simulink model "Model_xspmono_csa_ga"  (R2017a)
settings: Solver=ode45  StartTime=4.3  StopTime=9.196  MaxStep=0.001  RelTol=1e-3  AbsTol=1e-3  EnableMultiTasking=on
values from neighbouring files (symbols this model uses):
  F1 = F(1:11)    [Plot_results_last.m]
  K1_csa_ga = 2.26205318539721    (= 2.2620531854)    [Plot_results_last.m]
  K5_csa_ga = 1.94337888356766    (= 1.94337888357)    [Plot_results_last.m]
  Ks_csa_ga = 0.00300000000000    (= 0.003)    [Plot_results_last.m]
  Mmax_csa_ga = 0.90000000000000    (= 0.9)    [Plot_results_last.m]
  P0 = P1(1)    [Plot_results_last.m]
  Sd = [Sdop; Sd1]    [Plot_results_last.m]
  So = 500    [Plot_results_last.m]
  t1 = t(1:11)    [Plot_results_last.m]
  V1 = V(1:11)    [Plot_results_last.m]
  Xd = [Xdop; Xd1]    [Plot_results_last.m]
settings Model: ExtModeTrigMode=oneshot  ExtModeArmWhenConnect=off  Creator=i7_Pc  LastModifiedBy=i7_Pc
settings DataIOCC: SaveFormat=Array  SignalLoggingSaveFormat=ModelDataLogs  SaveOutput=off  SaveTime=off
settings OptimizationCC: BlockReduction=off  BooleanDataType=off  ExpressionDepthLimit=2147483647  InitFltsAndDblsToZero=on  LifeSpan=inf
settings DebuggingCC: SaveWithParameterizedLinksMsg=none  UnderspecifiedInitializationDetection=Classic  MergeDetectMultiDrivingBlocksExec=none  SignalResolutionControl=TryResolveAllWithWarning  MultiTaskDSMMsg=warning  MultiTaskCondExecSysMsg=none  FcnCallInpInsideContextMsg=warning  StateNameClashWarn=warning  SFUnexpectedBacktrackingDiag=warning  SFNoUnconditionalDefaultTransitionDiag=warning  SFExecutionAtInitializationDiag=none
settings HardwareCC: ProdBitPerPointer=32  ProdBitPerSizeT=32  ProdBitPerPtrDiffT=32  ProdLargestAtomicFloat=None  ProdIntDivRoundTo=Undefined  ProdEndianess=Unspecified  ProdWordSize=32  ProdHWDeviceType=32-bit Generic  TargetUnknown=on
settings ModelReferenceCC: PropagateSignalLabelsOutOfModel=off
settings GRTTargetCC: TargetLangStandard=C89/C90 (ANSI)  GeneratePreprocessorConditionals=Disable all  CombineOutputUpdateFcns=off  GRTInterface=on
settings ConfigComp: CovMetricSettings=dw  CovHtmlReporting=on  CovSaveCumulativeToWorkspaceVar=on  CovSaveSingleToWorkspaceVar=on  CovExternalEMLEnable=off

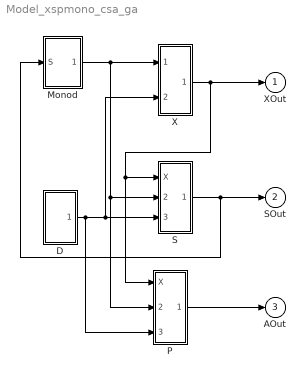
== system Model_xspmono_csa_ga ==
  D : Subsystem
  Monod : Subsystem
  P : Subsystem
  S : Subsystem
  X : Subsystem
  XOut : Outport
  SOut : Outport  Port=2
  AOut : Outport  Port=3
  wires:
  X/1(XOut) -> S/1(X), P/1(X), XOut/1
  S/1(Sout) -> Monod/1(S), SOut/1
  Monod/1(mu) -> X/1(mu), S/2(mu), P/2(mu)
  D/1(out_1) -> S/3(F/V), X/2(F/V), P/3(F/V)
  P/1(Pout) -> AOut/1

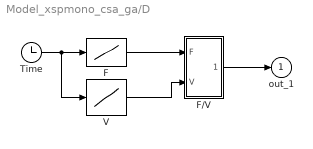
== system Model_xspmono_csa_ga/D ==
  F : Lookup  InputValues=t1  Table=F1  SaturateOnIntegerOverflow=on
  F/V : Subsystem  mask(/){}
      mask help: Division of two scalars. y=u[1]/u[2]
      mask Help: Division of two scalars: y=u[1]/u[2]
      mask Display: disp('/')
  Time : Clock
  V : Lookup  InputValues=t1  Table=V1  SaturateOnIntegerOverflow=on
  out_1 : Outport
  wires:
  F/V/1(out_1) -> out_1/1
  F/1 -> F/V/1(F)
  V/1 -> F/V/2(V)
  Time/1 -> F/1, V/1

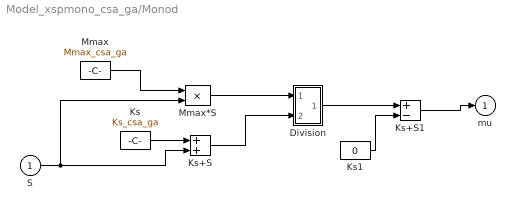
== system Model_xspmono_csa_ga/Monod ==
  S : Inport
  Division : Subsystem  mask(/){}
      mask help: Division of two scalars. y=u[1]/u[2]
      mask Help: Division of two scalars: y=u[1]/u[2]
      mask Display: disp('/')
  Ks : Constant  Value=Ks_csa_ga
  Ks+S : Sum  SaturateOnIntegerOverflow=on  InputSameDT=on  OutDataTypeStr=Inherit: Same as first input
  Ks+S1 : Sum  Inputs=+-  SaturateOnIntegerOverflow=on  InputSameDT=on  OutDataTypeStr=Inherit: Same as first input
  Ks1 : Constant  Value=0
  Mmax : Constant  Value=Mmax_csa_ga
  Mmax*S : Product  SaturateOnIntegerOverflow=on  RndMeth=Zero  InputSameDT=on  OutDataTypeStr=Inherit: Same as first input
  mu : Outport
  wires:
  Mmax/1 -> Mmax*S/1
  Mmax*S/1 -> Division/1(Mmax*S)
  Ks+S/1 -> Division/2(Ks+S)
  Ks/1 -> Ks+S/1
  S/1 -> Ks+S/2, Mmax*S/2
  Division/1(out_1) -> Ks+S1/1
  Ks1/1 -> Ks+S1/2
  Ks+S1/1 -> mu/1

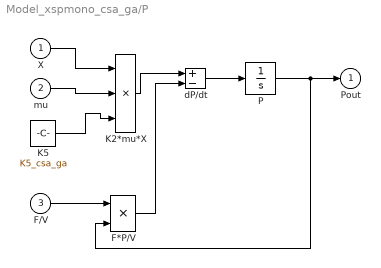
== system Model_xspmono_csa_ga/P ==
  X : Inport
  mu : Inport  Port=2
  F/V : Inport  Port=3
  F*P/V : Product  SaturateOnIntegerOverflow=on  RndMeth=Zero  InputSameDT=on  OutDataTypeStr=Inherit: Same as first input
  K2*mu*X : Product  Inputs=3  SaturateOnIntegerOverflow=on  RndMeth=Zero  InputSameDT=on  OutDataTypeStr=Inherit: Same as first input
  K5 : Constant  Value=K5_csa_ga
  P : Integrator  InitialCondition=P0
  dP/dt : Sum  Inputs=+-  SaturateOnIntegerOverflow=on  InputSameDT=on  OutDataTypeStr=Inherit: Same as first input
  Pout : Outport
  wires:
  P/1 -> Pout/1, F*P/V/2
  dP/dt/1 -> P/1
  K2*mu*X/1 -> dP/dt/1
  X/1 -> K2*mu*X/1
  mu/1 -> K2*mu*X/2
  F/V/1 -> F*P/V/1
  F*P/V/1 -> dP/dt/2
  K5/1 -> K2*mu*X/3

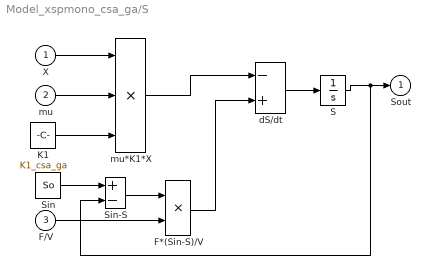
== system Model_xspmono_csa_ga/S ==
  X : Inport
  mu : Inport  Port=2
  F/V : Inport  Port=3
  F*(Sin-S)/V : Product  SaturateOnIntegerOverflow=on  RndMeth=Zero  InputSameDT=on  OutDataTypeStr=Inherit: Same as first input
  K1 : Constant  Value=K1_csa_ga
  S : Integrator  InitialCondition=Sd(1)  UpperSaturationLimit=1000  LowerSaturationLimit=0
  Sin : Constant  Value=So
  Sin-S : Sum  Inputs=+-  SaturateOnIntegerOverflow=on  InputSameDT=on  OutDataTypeStr=Inherit: Same as first input
  dS/dt : Sum  Inputs=-+  SaturateOnIntegerOverflow=on  InputSameDT=on  OutDataTypeStr=Inherit: Same as first input
  mu*K1*X : Product  Inputs=3  SaturateOnIntegerOverflow=on  RndMeth=Zero  InputSameDT=on  OutDataTypeStr=Inherit: Same as first input
  Sout : Outport
  wires:
  S/1 -> Sout/1, Sin-S/2
  Sin-S/1 -> F*(Sin-S)/V/1
  Sin/1 -> Sin-S/1
  X/1 -> mu*K1*X/1
  F/V/1 -> F*(Sin-S)/V/2
  mu*K1*X/1 -> dS/dt/1
  F*(Sin-S)/V/1 -> dS/dt/2
  dS/dt/1 -> S/1
  mu/1 -> mu*K1*X/2
  K1/1 -> mu*K1*X/3

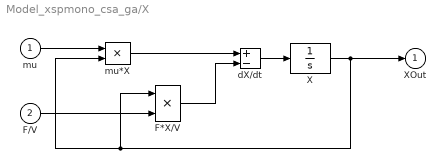
== system Model_xspmono_csa_ga/X ==
  mu : Inport
  F/V : Inport  Port=2
  F*X/V : Product  SaturateOnIntegerOverflow=on  RndMeth=Zero  InputSameDT=on  OutDataTypeStr=Inherit: Same as first input
  X : Integrator  InitialCondition=Xd(1)  UpperSaturationLimit=1000  LowerSaturationLimit=0
  dX/dt : Sum  Inputs=+-  SaturateOnIntegerOverflow=on  InputSameDT=on  OutDataTypeStr=Inherit: Same as first input
  mu*X : Product  SaturateOnIntegerOverflow=on  RndMeth=Zero  InputSameDT=on  OutDataTypeStr=Inherit: Same as first input
  XOut : Outport
  wires:
  F*X/V/1 -> dX/dt/2
  dX/dt/1 -> X/1
  mu*X/1 -> dX/dt/1
  mu/1 -> mu*X/1
  X/1 -> XOut/1, mu*X/2, F*X/V/1
  F/V/1 -> F*X/V/2

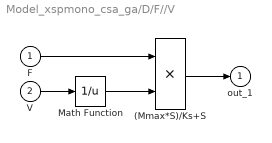
== system Model_xspmono_csa_ga/D/F//V ==
  F : Inport
  V : Inport  Port=2
  (Mmax*S)/Ks+S : Product  SaturateOnIntegerOverflow=on  RndMeth=Zero  InputSameDT=on  OutDataTypeStr=Inherit: Same as first input
  Math Function : Math  Operator=reciprocal  SaturateOnIntegerOverflow=on
  out_1 : Outport
  wires:
  F/1 -> (Mmax*S)/Ks+S/1
  V/1 -> Math Function/1
  Math Function/1 -> (Mmax*S)/Ks+S/2
  (Mmax*S)/Ks+S/1 -> out_1/1

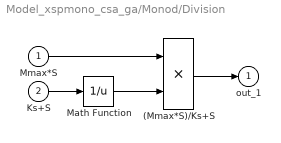
== system Model_xspmono_csa_ga/Monod/Division ==
  Mmax*S : Inport
  Ks+S : Inport  Port=2
  (Mmax*S)/Ks+S : Product  SaturateOnIntegerOverflow=on  RndMeth=Zero  InputSameDT=on  OutDataTypeStr=Inherit: Same as first input
  Math Function : Math  Operator=reciprocal  SaturateOnIntegerOverflow=on
  out_1 : Outport
  wires:
  Mmax*S/1 -> (Mmax*S)/Ks+S/1
  Ks+S/1 -> Math Function/1
  Math Function/1 -> (Mmax*S)/Ks+S/2
  (Mmax*S)/Ks+S/1 -> out_1/1
